simulink model "InverterModel"  (R2016a)
settings: Solver=FixedStepDiscrete  StartTime=0.0  StopTime=0.55e-6  FixedStep=SampleTime  RelTol=1e-3
values from neighbouring files (symbols this model uses):
  DelayTop = 0    [InverterMFile.m]
  Dtop = 48    [InverterMFile.m]
  fsw = 2000e3    (= 2000000)    [InverterMFile.m]
  Rd = 0.0024 + 1e-4    (= 0.0025)    [InverterMFile.m]
  Rg = 1.5    [InverterMFile.m]
  Rload = 20    [InverterMFile.m]    (also in TwoLevelSPWM-Hakan.m = Zload*Load_Power_Factor)
  Roff = 2    [InverterMFile.m]
  Ron = 15    [InverterMFile.m]
  Rs = 0.0433 + 1e-4    (= 0.0434)    [InverterMFile.m]
  Rss = 1e-3    (= 0.001)    [InverterMFile.m]
  VpulseMax = 6    [InverterMFile.m]
  VpulseMin = -3    [InverterMFile.m]
libraries: elec_lib x129, nesl_utility x91, fl_lib x80, simulink x6
(part 3 of 5)

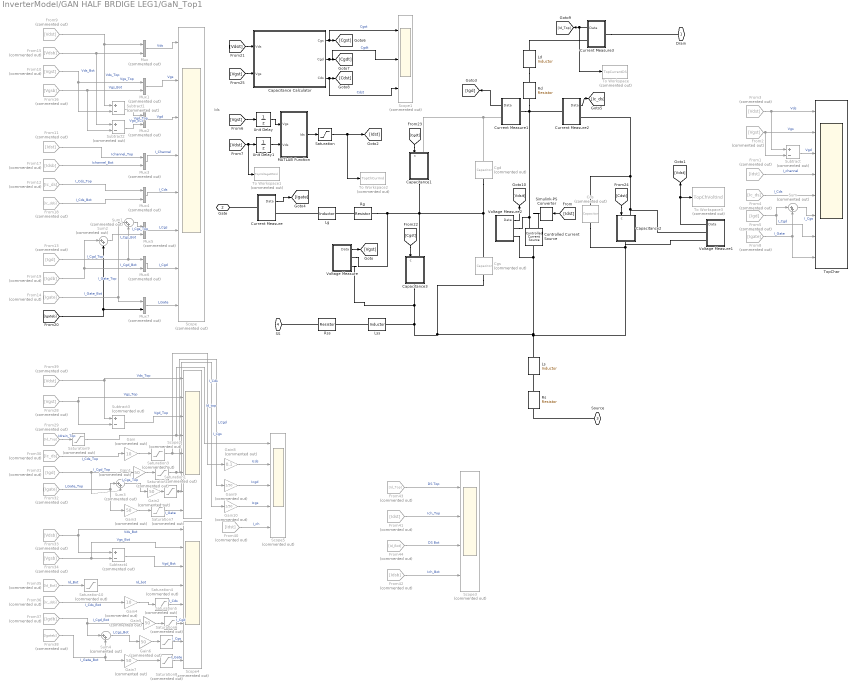
== system InverterModel/GAN HALF BRDIGE LEG1/GaN_Top1 ==
  note: Ids
  Capacitance Calculator : Subsystem
  Capacitance1 : Subsystem
  Capacitance2 : Subsystem
  Capacitance3 : Subsystem
  Cds : elec_lib/Passive Devices/Capacitor  Commented=on  enable_table=0  c=Cds F  Cvec=[ 1e-5 1e-6 ] F  Vvec=[ 0 10 ] V  CV_table_symmetry=1  C_tol=5  enable_C_tol=0  tol_distribution=1  nSigma=4  r=1e-6 Ohm  g=0 1/Ohm  initV=Vdc V  enable_operating_limits=0  operating_limit_action=2  max_working_voltage_range=[ -25 25 ] V  power_rating=1 W  enable_faults=0  fault_action=1  Cscale_faulted=100  R_faulted=0.001 Ohm  G_faulted=0 1/Ohm  tau_fault=0.001 s  enable_temporal_fault=0  t_fault=1 s  enable_behavioral_fault=0  max_permissible_voltage_range=[ -100 100 ] V  t_fail_on_voltage=1 s
  Cgd : elec_lib/Passive Devices/Capacitor  Commented=on  enable_table=0  c=Cgd F  Cvec=[ 1e-5 1e-6 ] F  Vvec=[ 0 10 ] V  CV_table_symmetry=1  C_tol=5  enable_C_tol=0  tol_distribution=1  nSigma=4  r=1e-6 Ohm  g=0 1/Ohm  initV=-VpulseMax V  enable_operating_limits=0  operating_limit_action=2  max_working_voltage_range=[ -25 25 ] V  power_rating=1 W  enable_faults=0  fault_action=1  Cscale_faulted=100  R_faulted=0.001 Ohm  G_faulted=0 1/Ohm  tau_fault=0.001 s  enable_temporal_fault=0  t_fault=1 s  enable_behavioral_fault=0  max_permissible_voltage_range=[ -100 100 ] V  t_fail_on_voltage=1 s
  Cgs : elec_lib/Passive Devices/Capacitor  Commented=on  enable_table=0  c=Cgs F  Cvec=[ 1e-5 1e-6 ] F  Vvec=[ 0 10 ] V  CV_table_symmetry=1  C_tol=5  enable_C_tol=0  tol_distribution=1  nSigma=4  r=1e-6 Ohm  g=0 1/Ohm  initV=VpulseMin V  enable_operating_limits=0  operating_limit_action=2  max_working_voltage_range=[ -25 25 ] V  power_rating=1 W  enable_faults=0  fault_action=1  Cscale_faulted=100  R_faulted=0.001 Ohm  G_faulted=0 1/Ohm  tau_fault=0.001 s  enable_temporal_fault=0  t_fault=1 s  enable_behavioral_fault=0  max_permissible_voltage_range=[ -100 100 ] V  t_fail_on_voltage=1 s
  Controlled Current Source : fl_lib/Electrical/Electrical Sources/Controlled Current Source
  Current Measure : Subsystem
  Current Measure1 : Subsystem
  Current Measure2 : Subsystem
  Current Measure3 : Subsystem
  From{1,11,40..41} (4 alike) : From  Commented=on  GotoTag=Idst  TagVisibility=global
  From10 : From  Commented=on  GotoTag=Vgst  TagVisibility=global
  From12 : From  Commented=on  GotoTag=Ic_ds
  From13 : From  Commented=on  GotoTag=Igd
  From14 : From  Commented=on  GotoTag=Igate
  From15 : From  Commented=on  GotoTag=Vdsb  TagVisibility=global
  From16 : From  Commented=on  GotoTag=Vgsb  TagVisibility=global
  From17 : From  Commented=on  GotoTag=Idsb  TagVisibility=global
  From18 : From  Commented=on  GotoTag=Ic_dsb  TagVisibility=global
  From19 : From  Commented=on  GotoTag=Igdb  TagVisibility=global
  From2 : From  Commented=on  GotoTag=Vgst  TagVisibility=global
  From28 : From  Commented=on  GotoTag=Vgst  TagVisibility=global
  From29 : From  Commented=on  GotoTag=Id_Top
  From3 : From  Commented=on  GotoTag=Vdst  TagVisibility=global
  From30 : From  Commented=on  GotoTag=Ic_ds
  From31 : From  Commented=on  GotoTag=Igd
  From32 : From  Commented=on  GotoTag=Igate
  From33 : From  Commented=on  GotoTag=Vdsb  TagVisibility=global
  From34 : From  Commented=on  GotoTag=Vgsb  TagVisibility=global
  From35 : From  Commented=on  GotoTag=Id_Bot  TagVisibility=global
  From36 : From  Commented=on  GotoTag=Ic_dsb  TagVisibility=global
  From37 : From  Commented=on  GotoTag=Igdb  TagVisibility=global
  From38 : From  Commented=on  GotoTag=Igateb  TagVisibility=global
  From39 : From  Commented=on  GotoTag=Vdst  TagVisibility=global
  From4 : From  Commented=on  GotoTag=Ic_ds
  From42 : From  Commented=on  GotoTag=Idsb  TagVisibility=global
  From43 : From  Commented=on  GotoTag=Id_Top
  From44 : From  Commented=on  GotoTag=Id_Bot  TagVisibility=global
  From5 : From  Commented=on  GotoTag=Igd
  From8 : From  Commented=on  GotoTag=Igate
  From9 : From  Commented=on  GotoTag=Vdst  TagVisibility=global
  Gain : Gain  Commented=on  Gain=10
  Gain{1..3,5..7} (6 alike) : Gain  Commented=on  Gain=50
  Gain10 : Gain  Commented=on  Gain=1/50
  Gain4 : Gain  Commented=on  Gain=10
  Gain8 : Gain  Commented=on  Gain=0.1
  Gain9 : Gain  Commented=on  Gain=1/50
  Ld : elec_lib/Passive Devices/Inductor  l=Ld H  L_tol=20  enable_L_tol=0  tol_distribution=1  nSigma=4  r=0 Ohm  g=1e-9 1/Ohm  initI=CurrBT A  enable_operating_limits=0  operating_limit_action=2  max_working_current=1 A  power_rating=1 W  enable_faults=0  fault_action=1  lambdaPercent=50  k_faulted=0.9999 Ohm  turnsShort=0  openCct=0  groundShort=0  groundShortG=0 1/Ohm  tau_fault=0.001 s  enable_temporal_fault=0  t_fault=1 s  enable_behavioral_fault=0  max_permissible_voltage=100 V  n_fail_on_voltage=1  max_permissible_current=1 A  t_fail_on_current=1 s
  Lg : elec_lib/Passive Devices/Inductor  l=Lg H  L_tol=20  enable_L_tol=0  tol_distribution=1  nSigma=4  r=0 Ohm  g=1e-9 1/Ohm  initI=0 A  enable_operating_limits=0  operating_limit_action=1  max_working_current=1 A  power_rating=1 W  enable_faults=0  fault_action=1  lambdaPercent=50  k_faulted=0.9999 Ohm  turnsShort=0  openCct=0  groundShort=0  groundShortG=0 1/Ohm  tau_fault=0.001 s  enable_temporal_fault=0  t_fault=1 s  enable_behavioral_fault=0  max_permissible_voltage=100 V  n_fail_on_voltage=1  max_permissible_current=1 A  t_fail_on_current=1 s
  Ls : elec_lib/Passive Devices/Inductor  l=Ls H  L_tol=20  enable_L_tol=0  tol_distribution=1  nSigma=4  r=0 Ohm  g=1e-9 1/Ohm  initI=CurrBT A  enable_operating_limits=0  operating_limit_action=2  max_working_current=1 A  power_rating=1 W  enable_faults=0  fault_action=1  lambdaPercent=50  k_faulted=0.9999 Ohm  turnsShort=0  openCct=0  groundShort=0  groundShortG=0 1/Ohm  tau_fault=0.001 s  enable_temporal_fault=0  t_fault=1 s  enable_behavioral_fault=0  max_permissible_voltage=100 V  n_fail_on_voltage=1  max_permissible_current=1 A  t_fail_on_current=1 s
  Lss : elec_lib/Passive Devices/Inductor  l=Lss H  L_tol=20  enable_L_tol=0  tol_distribution=1  nSigma=4  r=0 Ohm  g=1e-9 1/Ohm  initI=0 A  enable_operating_limits=0  operating_limit_action=2  max_working_current=1 A  power_rating=1 W  enable_faults=0  fault_action=1  lambdaPercent=50  k_faulted=0.9999 Ohm  turnsShort=0  openCct=0  groundShort=0  groundShortG=0 1/Ohm  tau_fault=0.001 s  enable_temporal_fault=0  t_fault=1 s  enable_behavioral_fault=0  max_permissible_voltage=100 V  n_fail_on_voltage=1  max_permissible_current=1 A  t_fail_on_current=1 s
  MATLAB Function : MATLAB Function  TreatAsAtomicUnit=on
  Mux{,1..7} (8 alike) : Mux  Commented=on  Inputs=2
  Rd : elec_lib/Passive Devices/Resistor  R=Rd Ohm  R_tol=5  enable_R_tol=0  tol_distribution=1  nSigma=4  enable_operating_limits=0  operating_limit_action=2  max_working_voltage=100 V  power_rating=1 W  enable_faults=0  fault_action=1  R_faulted=Inf Ohm  enable_temporal_fault=0  t_fault=1 s  enable_behavioral_fault=0  max_permissible_current=1 A  t_fail_on_current=1 s  noise_mode=0  sample_time=0.001 s  repeatability=1  auto_seed=2139298691  user_seed=0  Tdevice=25 degC  alpha=0.00393 1/K  Tmeas=25 degC  thermal_mass=100 J/K  initial_temperature=25 degC  power_derating_T1=70 degC  power_derating_T2=155 degC  operating_temperature_range_vec=[ -50 150 ] degC
  Rg : elec_lib/Passive Devices/Resistor  R=Rg Ohm  R_tol=5  enable_R_tol=0  tol_distribution=1  nSigma=4  enable_operating_limits=0  operating_limit_action=2  max_working_voltage=100 V  power_rating=1 W  enable_faults=0  fault_action=1  R_faulted=Inf Ohm  enable_temporal_fault=0  t_fault=1 s  enable_behavioral_fault=0  max_permissible_current=1 A  t_fail_on_current=1 s  noise_mode=0  sample_time=0.001 s  repeatability=1  auto_seed=3869131976  user_seed=0  Tdevice=25 degC  alpha=0.00393 1/K  Tmeas=25 degC  thermal_mass=100 J/K  initial_temperature=25 degC  power_derating_T1=70 degC  power_derating_T2=155 degC  operating_temperature_range_vec=[ -50 150 ] degC
  Rs : elec_lib/Passive Devices/Resistor  R=Rs Ohm  R_tol=5  enable_R_tol=0  tol_distribution=1  nSigma=4  enable_operating_limits=0  operating_limit_action=2  max_working_voltage=100 V  power_rating=1 W  enable_faults=0  fault_action=1  R_faulted=Inf Ohm  enable_temporal_fault=0  t_fault=1 s  enable_behavioral_fault=0  max_permissible_current=1 A  t_fail_on_current=1 s  noise_mode=0  sample_time=0.001 s  repeatability=1  auto_seed=2468151142  user_seed=0  Tdevice=25 degC  alpha=0.00393 1/K  Tmeas=25 degC  thermal_mass=100 J/K  initial_temperature=25 degC  power_derating_T1=70 degC  power_derating_T2=155 degC  operating_temperature_range_vec=[ -50 150 ] degC
  Rss : elec_lib/Passive Devices/Resistor  R=Rss Ohm  R_tol=5  enable_R_tol=0  tol_distribution=1  nSigma=4  enable_operating_limits=0  operating_limit_action=2  max_working_voltage=100 V  power_rating=1 W  enable_faults=0  fault_action=1  R_faulted=Inf Ohm  enable_temporal_fault=0  t_fault=1 s  enable_behavioral_fault=0  max_permissible_current=1 A  t_fail_on_current=1 s  noise_mode=0  sample_time=0.001 s  repeatability=1  auto_seed=3630012664  user_seed=0  Tdevice=25 degC  alpha=0.00393 1/K  Tmeas=25 degC  thermal_mass=100 J/K  initial_temperature=25 degC  power_derating_T1=70 degC  power_derating_T2=155 degC  operating_temperature_range_vec=[ -50 150 ] degC
  Saturation : Saturate  UpperLimit=200  LowerLimit=-200
  Saturation{1..2,5..10} (8 alike) : Saturate  Commented=on  UpperLimit=100  LowerLimit=-100
  Saturation3 : Saturate  Commented=on  UpperLimit=250  LowerLimit=-100
  Saturation4 : Saturate  Commented=on  UpperLimit=250  LowerLimit=-100
  Scope : Scope  Commented=on  NumInputPorts=8
  Scope1 : Scope  Commented=on  NumInputPorts=3
  Scope2 : Scope  Commented=on  NumInputPorts=8
  Scope3 : Scope  Commented=on  NumInputPorts=4
  Scope4 : Scope  Commented=on  NumInputPorts=8
  Scope5 : Scope  Commented=on  NumInputPorts=5
  Simulink-PS Converter : nesl_utility/Simulink-PS Converter  PhysicalDomain=network_engine_domain  SubClassName=ps_input  LeftPortType=input  RightPortType=output  PseudoPeriodic=off  Frequencies=[]  NoiseDistribution=none  NoiseParameters=[]  Unit=1  AffineConversion=off  InputFiltering=off  SimscapeFilterOrder=1  InputFilterTimeConstant=0.001  UdotUserProvided=1
  Subtract{,1..4} (5 alike) : Sum  Commented=on  Inputs=+-
  Sum{,1..4} (5 alike) : Sum  Commented=on  Inputs=|++
  To Workspace : ToWorkspace  Commented=on  VariableName=TopCurrentDS  SampleTime=-1
      settings: Save2DSignal=2-D array (concatenate along first dimension)
  To Workspace1 : ToWorkspace  Commented=on  VariableName=TopVoltageDSInd  SampleTime=-1
      settings: Save2DSignal=2-D array (concatenate along first dimension)
  To Workspace2 : ToWorkspace  Commented=on  VariableName=TopChCurrInd  SampleTime=-1
      settings: Save2DSignal=2-D array (concatenate along first dimension)
  To Workspace3 : ToWorkspace  Commented=on  VariableName=TopChVoltInd  SampleTime=-1
      settings: Save2DSignal=2-D array (concatenate along first dimension)
  TopChar : Scope  NumInputPorts=8
  Unit Delay : UnitDelay  SampleTime=-1
  Unit Delay1 : UnitDelay  SampleTime=-1
  Voltage Measure : Subsystem
  Voltage Measure1 : Subsystem
  Voltage Measure2 : Subsystem
  Drain : PMIOPort  Port=1  Side=Right
  Gate : PMIOPort  Port=2  Side=Left
  Source : PMIOPort  Port=3  Side=Right
  SS : PMIOPort  Port=4  Side=Left
  wires:
  [Vgst] -> Capacitance Calculator/2(Vgs)
  From44/1 -> Scope3/3  "DS Bot"
  From43/1 -> Scope3/1  "DS Top"
  Voltage Measure1/1(Data) -> [Vdst], To Workspace3/1
  Saturation/1 -> To Workspace2/1, [Idst]
  Voltage Measure2/1(Data) -> [Vdsit]
  Unit Delay1/1 -> MATLAB Function/2(Vds)
  [Vdst] -> To Workspace1/1, Unit Delay1/1
  From42/1 -> Scope3/4  "Ich_Bot"
  From41/1 -> Scope3/2  "Ich_Top"
  From40/1 -> Scope5/5  "I_ch"
  Gain10/1 -> Scope5/4  "Icgs"
  Gain9/1 -> Scope5/3  "Icgd"
  Gain8/1 -> Scope5/2  "Icds"
  Saturation10/1 -> Scope4/4  "Id_bot"
  Saturation9/1 -> Scope2/4, Scope5/1  "Id_top"
  Current Measure3/1(Data) -> [Id_Top], To Workspace/1
  Saturation8/1 -> Scope4/8  "I_Gate"
  Saturation7/1 -> Scope2/8  "I_Gate"
  Saturation6/1 -> Scope4/7  "I_Cgs"
  Gain5/1 -> Saturation5/1
  Saturation5/1 -> Scope4/6  "I_Cgd"
  Saturation4/1 -> Scope4/5  "I_Cds"
  Saturation3/1 -> Scope2/5, Gain8/1  "I_Cds"
  Saturation2/1 -> Scope2/6, Gain9/1  "I_Cgd"
  Saturation1/1 -> Scope2/7, Gain10/1  "I_Cgs"
  Gain2/1 -> Saturation1/1
  Gain7/1 -> Saturation8/1
  Gain6/1 -> Saturation6/1
  Gain4/1 -> Saturation4/1
  Gain3/1 -> Saturation7/1
  Sum3/1 -> Gain2/1  "I_Cgs_Top"
  Gain1/1 -> Saturation2/1
  Gain/1 -> Saturation3/1
  Sum4/1 -> Gain6/1  "I_Cgs_Bot"
  From35/1 -> Saturation10/1  "Id_Bot"
  From29/1 -> Saturation9/1  "Idrain_Top"
  Subtract4/1 -> Scope4/3  "Vgd_Bot"
  Subtract3/1 -> Scope2/3  "Vgd_Top"
  From38/1 -> Sum4/2, Gain7/1  "I_Gate_Bot"
  From37/1 -> Gain5/1, Sum4/1  "I_Cgd_Bot"
  From36/1 -> Gain4/1  "I_Cds_Bot"
  From34/1 -> Subtract4/2, Scope4/2  "Vgs_Bot"
  From33/1 -> Subtract4/1, Scope4/1  "Vds_Bot"
  From32/1 -> Sum3/1, Gain3/1  "I_Gate_Top"
  From31/1 -> Gain1/1, Sum3/2  "I_Cgd_Top"
  From30/1 -> Gain/1  "I_Cds_Top"
  From28/1 -> Subtract3/2, Scope2/2  "Vgs_Top"
  From39/1 -> Subtract3/1, Scope2/1  "Vds_Top"
  [Cdst] -> Capacitance2/1(c)
  [Cgdt] -> Capacitance1/1(c)
  [Cgst] -> Capacitance3/1(c)
  Capacitance Calculator/3(Cds) -> [Cdst], Scope1/3  "Cdst"
  Capacitance Calculator/2(Cgd) -> [Cgdt], Scope1/2  "Cgdt"
  Capacitance Calculator/1(Cgs) -> [Cgst], Scope1/1  "Cgst"
  [Vdsit] -> Capacitance Calculator/1(Vds)
  Mux/1 -> Scope/1  "Vds"
  Mux1/1 -> Scope/2  "Vgs"
  Mux2/1 -> Scope/3  "Vgd"
  Mux3/1 -> Scope/4  "I_Channel"
  Mux4/1 -> Scope/5  "I_Cds"
  Mux5/1 -> Scope/6  "I_Cgs"
  Mux6/1 -> Scope/7  "I_Cgd"
  Mux7/1 -> Scope/8  "I_Gate"
  From17/1 -> Mux3/2  "Ichannel_Bot"
  From11/1 -> Mux3/1  "Ichannel_Top"
  Subtract2/1 -> Mux2/2  "Vgd_Bot"
  Subtract1/1 -> Mux2/1  "Vgd_Top"
  Sum2/1 -> Mux5/2  "I_Cgs_Bot"
  [Igateb] -> Sum2/2, Mux7/2  "I_Gate_Bot"
  From19/1 -> Sum2/1, Mux6/2  "I_Cgd_Bot"
  From18/1 -> Mux4/2  "I_Cds_Bot"
  From16/1 -> Subtract2/2, Mux1/2  "Vgs_Bot"
  From15/1 -> Mux/2, Subtract2/1  "Vds_Bot"
  Sum1/1 -> Mux5/1  "I_Cgs_Top"
  From14/1 -> Sum1/1, Mux7/1  "I_Gate_Top"
  From13/1 -> Sum1/2, Mux6/1  "I_Cgd_Top"
  From12/1 -> Mux4/1  "I_Cds_Top"
  From10/1 -> Subtract1/2, Mux1/1  "Vgs_Top"
  From9/1 -> Subtract1/1, Mux/1  "Vds_Top"
  Voltage Measure/1(Data) -> [Vgst]
  Current Measure/1(Data) -> [Igate]
  Sum/1 -> TopChar/6  "I_Cgs"
  From4/1 -> TopChar/5  "I_Cds"
  From8/1 -> Sum/2, TopChar/8  "I_Gate"
  From5/1 -> Sum/1, TopChar/7  "I_Cgd"
  Current Measure2/1(Data) -> [Ic_ds]
  Current Measure1/1(Data) -> [Igd]
  Subtract/1 -> TopChar/3  "Vgd"
  From1/1 -> TopChar/4  "I_channel"
  From3/1 -> TopChar/1, Subtract/1  "Vds"
  From2/1 -> TopChar/2, Subtract/2  "Vgs"
  [Idst] -> Simulink-PS Converter/1
  Unit Delay/1 -> MATLAB Function/1(Vgs)
  MATLAB Function/1(Ids) -> Saturation/1
  [Vgst] -> Unit Delay/1
  connections:
  Rg/RConn1 -- Lg/RConn1
  Current Measure3/RConn1 -- Ld/LConn1
  Rs/LConn1 -- Ls/RConn1
  Lss/LConn1 -- Rss/RConn1
  Ld/RConn1 -- Rd/LConn1
  Source/RConn1 -- Rs/RConn1
  Voltage Measure/RConn2 -- Capacitance3/RConn1 -- Cgs/RConn1 -- Voltage Measure2/RConn2 -- Controlled Current Source/LConn1 -- Capacitance2/RConn1 -- Voltage Measure1/RConn2 -- Cds/RConn1 -- Ls/LConn1 -- Lss/RConn1
  Rss/LConn1 -- SS/RConn1
  Lg/LConn1 -- Current Measure/RConn1
  Current Measure1/LConn1 -- Rd/RConn1 -- Controlled Current Source/RConn2 -- Voltage Measure2/RConn1 -- Current Measure2/LConn1
  Current Measure3/LConn1 -- Drain/RConn1
  Current Measure2/RConn1 -- Cds/LConn1 -- Voltage Measure1/RConn1 -- Capacitance2/LConn1
  Cgd/LConn1 -- Current Measure1/RConn1 -- Capacitance1/LConn1
  Current Measure/LConn1 -- Gate/RConn1
  Simulink-PS Converter/RConn1 -- Controlled Current Source/RConn1
  Voltage Measure/RConn1 -- Rg/LConn1 -- Capacitance3/LConn1 -- Cgd/RConn1 -- Cgs/LConn1 -- Capacitance1/RConn1

== system InverterModel/GAN HALF BRDIGE LEG1/Voltage Measure3 ==
  PS-Simulink Converter2 : nesl_utility/PS-Simulink Converter  PhysicalDomain=network_engine_domain  SubClassName=ps_output  LeftPortType=input  RightPortType=output  PseudoPeriodic=off  Frequencies=[]  Unit=1  AffineConversion=off
  Voltage Sensor3 : fl_lib/Electrical/Electrical Sensors/Voltage Sensor
  V+ : PMIOPort  Port=1  Side=Right
  V- : PMIOPort  Port=2  Side=Right
  Data : Outport
  wires:
  PS-Simulink Converter2/1 -> Data/1
  connections:
  PS-Simulink Converter2/LConn1 -- Voltage Sensor3/RConn1
  Voltage Sensor3/RConn2 -- V-/RConn1
  Voltage Sensor3/LConn1 -- V+/RConn1

== system InverterModel/GAN HALF BRDIGE LEG1/Voltage Measure6 ==
  PS-Simulink Converter2 : nesl_utility/PS-Simulink Converter  PhysicalDomain=network_engine_domain  SubClassName=ps_output  LeftPortType=input  RightPortType=output  PseudoPeriodic=off  Frequencies=[]  Unit=1  AffineConversion=off
  Voltage Sensor3 : fl_lib/Electrical/Electrical Sensors/Voltage Sensor
  V+ : PMIOPort  Port=1  Side=Right
  V- : PMIOPort  Port=2  Side=Right
  Data : Outport
  wires:
  PS-Simulink Converter2/1 -> Data/1
  connections:
  Voltage Sensor3/LConn1 -- V+/RConn1
  Voltage Sensor3/RConn2 -- V-/RConn1
  PS-Simulink Converter2/LConn1 -- Voltage Sensor3/RConn1

== system InverterModel/GAN HALF BRDIGE LEG2/Current Measure4 ==
  Current Sensor1 : fl_lib/Electrical/Electrical Sensors/Current Sensor
  PS-Simulink Converter4 : nesl_utility/PS-Simulink Converter  PhysicalDomain=network_engine_domain  SubClassName=ps_output  LeftPortType=input  RightPortType=output  PseudoPeriodic=off  Frequencies=[]  Unit=1  AffineConversion=off
  I+ : PMIOPort  Port=1  Side=Left
  I- : PMIOPort  Port=2  Side=Right
  Data : Outport
  wires:
  PS-Simulink Converter4/1 -> Data/1
  connections:
  Current Sensor1/LConn1 -- I+/RConn1
  PS-Simulink Converter4/LConn1 -- Current Sensor1/RConn1
  Current Sensor1/RConn2 -- I-/RConn1

== system InverterModel/GAN HALF BRDIGE LEG2/Current Measure5 ==
  Current Sensor1 : fl_lib/Electrical/Electrical Sensors/Current Sensor
  PS-Simulink Converter4 : nesl_utility/PS-Simulink Converter  PhysicalDomain=network_engine_domain  SubClassName=ps_output  LeftPortType=input  RightPortType=output  PseudoPeriodic=off  Frequencies=[]  Unit=1  AffineConversion=off
  I+ : PMIOPort  Port=1  Side=Left
  I- : PMIOPort  Port=2  Side=Right
  Data : Outport
  wires:
  PS-Simulink Converter4/1 -> Data/1
  connections:
  Current Sensor1/RConn2 -- I-/RConn1
  PS-Simulink Converter4/LConn1 -- Current Sensor1/RConn1
  Current Sensor1/LConn1 -- I+/RConn1

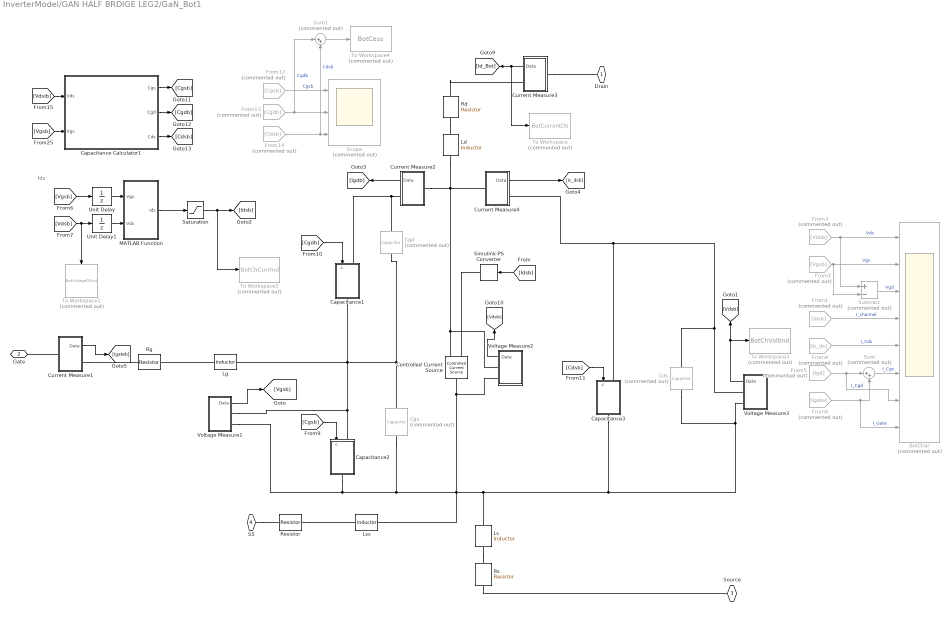
== system InverterModel/GAN HALF BRDIGE LEG2/GaN_Bot1 ==
  note: Ids
  BotChar : Scope  Commented=on  NumInputPorts=8
  Capacitance Calculator1 : Subsystem
  Capacitance1 : Subsystem
  Capacitance2 : Subsystem
  Capacitance3 : Subsystem
  Cds : elec_lib/Passive Devices/Capacitor  Commented=on  enable_table=0  c=Cds F  Cvec=[ 1e-5 1e-6 ] F  Vvec=[ 0 10 ] V  CV_table_symmetry=1  C_tol=5  enable_C_tol=0  tol_distribution=1  nSigma=4  r=1e-6 Ohm  g=0 1/Ohm  initV=0 V  enable_operating_limits=0  operating_limit_action=2  max_working_voltage_range=[ -25 25 ] V  power_rating=1 W  enable_faults=0  fault_action=1  Cscale_faulted=100  R_faulted=0.001 Ohm  G_faulted=0 1/Ohm  tau_fault=0.001 s  enable_temporal_fault=0  t_fault=1 s  enable_behavioral_fault=0  max_permissible_voltage_range=[ -100 100 ] V  t_fail_on_voltage=1 s
  Cgd : elec_lib/Passive Devices/Capacitor  Commented=on  enable_table=0  c=Cgd F  Cvec=[ 1e-5 1e-6 ] F  Vvec=[ 0 10 ] V  CV_table_symmetry=1  C_tol=5  enable_C_tol=0  tol_distribution=1  nSigma=4  r=1e-6 Ohm  g=0 1/Ohm  initV=Vdc - VpulseMin V  enable_operating_limits=0  operating_limit_action=2  max_working_voltage_range=[ -25 25 ] V  power_rating=1 W  enable_faults=0  fault_action=1  Cscale_faulted=100  R_faulted=0.001 Ohm  G_faulted=0 1/Ohm  tau_fault=0.001 s  enable_temporal_fault=0  t_fault=1 s  enable_behavioral_fault=0  max_permissible_voltage_range=[ -100 100 ] V  t_fail_on_voltage=1 s
  Cgs : elec_lib/Passive Devices/Capacitor  Commented=on  enable_table=0  c=Cgs F  Cvec=[ 1e-5 1e-6 ] F  Vvec=[ 0 10 ] V  CV_table_symmetry=1  C_tol=5  enable_C_tol=0  tol_distribution=1  nSigma=4  r=1e-6 Ohm  g=0 1/Ohm  initV=VpulseMax V  enable_operating_limits=0  operating_limit_action=2  max_working_voltage_range=[ -25 25 ] V  power_rating=1 W  enable_faults=0  fault_action=1  Cscale_faulted=100  R_faulted=0.001 Ohm  G_faulted=0 1/Ohm  tau_fault=0.001 s  enable_temporal_fault=0  t_fault=1 s  enable_behavioral_fault=0  max_permissible_voltage_range=[ -100 100 ] V  t_fail_on_voltage=1 s
  Controlled Current Source : fl_lib/Electrical/Electrical Sources/Controlled Current Source
  Current Measure1 : Subsystem
  Current Measure2 : Subsystem
  Current Measure3 : Subsystem
  Current Measure4 : Subsystem
  From1 : From  Commented=on  GotoTag=Idsb  TagVisibility=global
  From12 : From  Commented=on  GotoTag=Cgsb
  From13 : From  Commented=on  GotoTag=Cgdb
  From14 : From  Commented=on  GotoTag=Cdsb
  From2 : From  Commented=on  GotoTag=Vgsb  TagVisibility=global
  From3 : From  Commented=on  GotoTag=Vdsb  TagVisibility=global
  From4 : From  Commented=on  GotoTag=Ic_ds
  From5 : From  Commented=on  GotoTag=Igd
  From8 : From  Commented=on  GotoTag=Igate
  Ld : elec_lib/Passive Devices/Inductor  l=Ld H  L_tol=20  enable_L_tol=0  tol_distribution=1  nSigma=4  r=0 Ohm  g=1e-9 1/Ohm  initI=CurrCB A  enable_operating_limits=0  operating_limit_action=2  max_working_current=1 A  power_rating=1 W  enable_faults=0  fault_action=1  lambdaPercent=50  k_faulted=0.9999 Ohm  turnsShort=0  openCct=0  groundShort=0  groundShortG=0 1/Ohm  tau_fault=0.001 s  enable_temporal_fault=0  t_fault=1 s  enable_behavioral_fault=0  max_permissible_voltage=100 V  n_fail_on_voltage=1  max_permissible_current=1 A  t_fail_on_current=1 s
  "Lg " : elec_lib/Passive Devices/Inductor  l=Lg H  L_tol=20  enable_L_tol=0  tol_distribution=1  nSigma=4  r=0 Ohm  g=1e-9 1/Ohm  initI=0 A  enable_operating_limits=0  operating_limit_action=2  max_working_current=1 A  power_rating=1 W  enable_faults=0  fault_action=1  lambdaPercent=50  k_faulted=0.9999 Ohm  turnsShort=0  openCct=0  groundShort=0  groundShortG=0 1/Ohm  tau_fault=0.001 s  enable_temporal_fault=0  t_fault=1 s  enable_behavioral_fault=0  max_permissible_voltage=100 V  n_fail_on_voltage=1  max_permissible_current=1 A  t_fail_on_current=1 s
  Ls : elec_lib/Passive Devices/Inductor  l=Ls H  L_tol=20  enable_L_tol=0  tol_distribution=1  nSigma=4  r=0 Ohm  g=1e-9 1/Ohm  initI=CurrCB A  enable_operating_limits=0  operating_limit_action=2  max_working_current=1 A  power_rating=1 W  enable_faults=0  fault_action=1  lambdaPercent=50  k_faulted=0.9999 Ohm  turnsShort=0  openCct=0  groundShort=0  groundShortG=0 1/Ohm  tau_fault=0.001 s  enable_temporal_fault=0  t_fault=1 s  enable_behavioral_fault=0  max_permissible_voltage=100 V  n_fail_on_voltage=1  max_permissible_current=1 A  t_fail_on_current=1 s
  Lss : elec_lib/Passive Devices/Inductor  l=Lss H  L_tol=20  enable_L_tol=0  tol_distribution=1  nSigma=4  r=0 Ohm  g=1e-9 1/Ohm  initI=0 A  enable_operating_limits=0  operating_limit_action=1  max_working_current=1 A  power_rating=1 W  enable_faults=0  fault_action=1  lambdaPercent=50  k_faulted=0.9999 Ohm  turnsShort=0  openCct=0  groundShort=0  groundShortG=0 1/Ohm  tau_fault=0.001 s  enable_temporal_fault=0  t_fault=1 s  enable_behavioral_fault=0  max_permissible_voltage=100 V  n_fail_on_voltage=1  max_permissible_current=1 A  t_fail_on_current=1 s
  MATLAB Function : MATLAB Function  TreatAsAtomicUnit=on
  Rd : elec_lib/Passive Devices/Resistor  R=Rd Ohm  R_tol=5  enable_R_tol=0  tol_distribution=1  nSigma=4  enable_operating_limits=0  operating_limit_action=2  max_working_voltage=100 V  power_rating=1 W  enable_faults=0  fault_action=1  R_faulted=Inf Ohm  enable_temporal_fault=0  t_fault=1 s  enable_behavioral_fault=0  max_permissible_current=1 A  t_fail_on_current=1 s  noise_mode=0  sample_time=0.001 s  repeatability=1  auto_seed=3172435897  user_seed=0  Tdevice=25 degC  alpha=0.00393 1/K  Tmeas=25 degC  thermal_mass=100 J/K  initial_temperature=25 degC  power_derating_T1=70 degC  power_derating_T2=155 degC  operating_temperature_range_vec=[ -50 150 ] degC
  Resistor : elec_lib/Passive Devices/Resistor  R=Rss Ohm  R_tol=5  enable_R_tol=0  tol_distribution=1  nSigma=4  enable_operating_limits=0  operating_limit_action=2  max_working_voltage=100 V  power_rating=1 W  enable_faults=0  fault_action=1  R_faulted=Inf Ohm  enable_temporal_fault=0  t_fault=1 s  enable_behavioral_fault=0  max_permissible_current=1 A  t_fail_on_current=1 s  noise_mode=0  sample_time=0.001 s  repeatability=1  auto_seed=2516795155  user_seed=0  Tdevice=25 degC  alpha=0.00393 1/K  Tmeas=25 degC  thermal_mass=100 J/K  initial_temperature=25 degC  power_derating_T1=70 degC  power_derating_T2=155 degC  operating_temperature_range_vec=[ -50 150 ] degC
  Rg : elec_lib/Passive Devices/Resistor  R=Rg Ohm  R_tol=5  enable_R_tol=0  tol_distribution=1  nSigma=4  enable_operating_limits=0  operating_limit_action=2  max_working_voltage=100 V  power_rating=1 W  enable_faults=0  fault_action=1  R_faulted=Inf Ohm  enable_temporal_fault=0  t_fault=1 s  enable_behavioral_fault=0  max_permissible_current=1 A  t_fail_on_current=1 s  noise_mode=0  sample_time=0.001 s  repeatability=1  auto_seed=1059716720  user_seed=0  Tdevice=25 degC  alpha=0.00393 1/K  Tmeas=25 degC  thermal_mass=100 J/K  initial_temperature=25 degC  power_derating_T1=70 degC  power_derating_T2=155 degC  operating_temperature_range_vec=[ -50 150 ] degC
  Rs : elec_lib/Passive Devices/Resistor  R=Rs Ohm  R_tol=5  enable_R_tol=0  tol_distribution=1  nSigma=4  enable_operating_limits=0  operating_limit_action=2  max_working_voltage=100 V  power_rating=1 W  enable_faults=0  fault_action=1  R_faulted=Inf Ohm  enable_temporal_fault=0  t_fault=1 s  enable_behavioral_fault=0  max_permissible_current=1 A  t_fail_on_current=1 s  noise_mode=0  sample_time=0.001 s  repeatability=1  auto_seed=2862235859  user_seed=0  Tdevice=25 degC  alpha=0.00393 1/K  Tmeas=25 degC  thermal_mass=100 J/K  initial_temperature=25 degC  power_derating_T1=70 degC  power_derating_T2=155 degC  operating_temperature_range_vec=[ -50 150 ] degC
  Saturation : Saturate  UpperLimit=200  LowerLimit=-200
  Scope : Scope  Commented=on  NumInputPorts=3
  Simulink-PS Converter : nesl_utility/Simulink-PS Converter  PhysicalDomain=network_engine_domain  SubClassName=ps_input  LeftPortType=input  RightPortType=output  PseudoPeriodic=off  Frequencies=[]  NoiseDistribution=none  NoiseParameters=[]  Unit=1  AffineConversion=off  InputFiltering=off  SimscapeFilterOrder=1  InputFilterTimeConstant=0.001  UdotUserProvided=1
  Subtract : Sum  Commented=on  Inputs=+-
  Sum : Sum  Commented=on  Inputs=|++
  Sum1 : Sum  Commented=on  Inputs=|++
  To Workspace : ToWorkspace  Commented=on  VariableName=BotCurrentDS  SampleTime=-1
      settings: Save2DSignal=2-D array (concatenate along first dimension)
  To Workspace1 : ToWorkspace  Commented=on  VariableName=BotVoltageDSInd  SampleTime=-1
      settings: Save2DSignal=2-D array (concatenate along first dimension)
  To Workspace2 : ToWorkspace  Commented=on  VariableName=BotChCurrInd  SampleTime=-1
      settings: Save2DSignal=2-D array (concatenate along first dimension)
  To Workspace3 : ToWorkspace  Commented=on  VariableName=BotChVoltInd  SampleTime=-1
      settings: Save2DSignal=2-D array (concatenate along first dimension)
  To Workspace4 : ToWorkspace  Commented=on  VariableName=BotCoss  SampleTime=-1
      settings: Save2DSignal=2-D array (concatenate along first dimension)
  Unit Delay : UnitDelay  SampleTime=-1
  Unit Delay1 : UnitDelay  SampleTime=-1
  Voltage Measure1 : Subsystem
  Voltage Measure2 : Subsystem
  Voltage Measure3 : Subsystem
  Drain : PMIOPort  Port=1  Side=Right
  Gate : PMIOPort  Port=2  Side=Left
  Source : PMIOPort  Port=3  Side=Right
  SS : PMIOPort  Port=4  Side=Left
  wires:
  Sum1/1 -> To Workspace4/1
  [Vgsb] -> Capacitance Calculator1/2(Vgs)
  Capacitance Calculator1/3(Cds) -> [Cdsb]
  Capacitance Calculator1/2(Cgd) -> [Cgdb]
  Capacitance Calculator1/1(Cgs) -> [Cgsb]
  [Vdsib] -> Capacitance Calculator1/1(Vds)
  Saturation/1 -> To Workspace2/1, [Idsb]
  Voltage Measure2/1(Data) -> [Vdsib]
  Unit Delay1/1 -> MATLAB Function/2(Vds)
  Current Measure3/1(Data) -> [Id_Bot], To Workspace/1
  From14/1 -> Scope/3, Sum1/2  "Cdsb"
  From13/1 -> Scope/2, Sum1/1  "Cgdb"
  From12/1 -> Scope/1  "Cgsb"
  [Cdsb] -> Capacitance3/1(c)
  [Cgdb] -> Capacitance1/1(c)
  [Cgsb] -> Capacitance2/1(c)
  Voltage Measure3/1(Data) -> [Vdsb], To Workspace3/1
  Current Measure1/1(Data) -> [Igateb]
  Sum/1 -> BotChar/6  "I_Cgs"
  Current Measure4/1(Data) -> [Ic_dsb]
  Current Measure2/1(Data) -> [Igdb]
  From8/1 -> Sum/2, BotChar/8  "I_Gate"
  From5/1 -> Sum/1, BotChar/7  "I_Cgd"
  From4/1 -> BotChar/5  "I_Cds"
  Subtract/1 -> BotChar/3  "Vgd"
  From1/1 -> BotChar/4  "I_channel"
  From3/1 -> Subtract/1, BotChar/1  "Vds"
  From2/1 -> Subtract/2, BotChar/2  "Vgs"
  [Idsb] -> Simulink-PS Converter/1
  [Vgsb] -> Unit Delay/1
  MATLAB Function/1(Ids) -> Saturation/1
  Unit Delay/1 -> MATLAB Function/1(Vgs)
  [Vdsb] -> To Workspace1/1, Unit Delay1/1
  Voltage Measure1/1(Data) -> [Vgsb]
  connections:
  Ls/RConn1 -- Rs/LConn1
  "Lg "/LConn1 -- Rg/LConn1
  Rd/RConn1 -- Ld/LConn1
  Resistor/RConn1 -- Lss/LConn1
  Rd/LConn1 -- Current Measure3/RConn1
  Rs/RConn1 -- Source/RConn1
  Voltage Measure3/RConn2 -- Cgs/RConn1 -- Capacitance2/RConn1 -- Voltage Measure1/RConn2 -- Voltage Measure2/RConn2 -- Controlled Current Source/LConn1 -- Lss/RConn1 -- Ls/LConn1 -- Capacitance3/RConn1 -- Cds/RConn1
  SS/RConn1 -- Resistor/LConn1
  Current Measure4/LConn1 -- Current Measure2/LConn1 -- Ld/RConn1 -- Voltage Measure2/RConn1 -- Controlled Current Source/RConn2
  Capacitance1/RConn1 -- Cgs/LConn1 -- Cgd/RConn1 -- "Lg "/RConn1 -- Voltage Measure1/RConn1 -- Capacitance2/LConn1
  Current Measure3/LConn1 -- Drain/RConn1
  Current Measure2/RConn1 -- Cgd/LConn1 -- Capacitance1/LConn1
  Current Measure1/RConn1 -- Rg/RConn1
  Current Measure4/RConn1 -- Capacitance3/LConn1 -- Cds/LConn1 -- Voltage Measure3/RConn1
  Current Measure1/LConn1 -- Gate/RConn1
  Simulink-PS Converter/RConn1 -- Controlled Current Source/RConn1

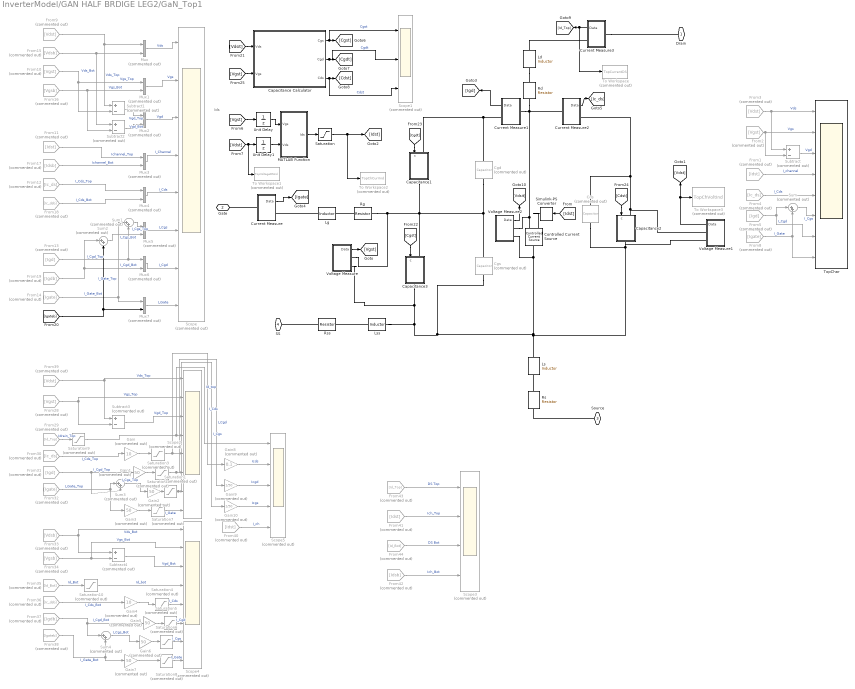
== system InverterModel/GAN HALF BRDIGE LEG2/GaN_Top1 ==
  note: Ids
  Capacitance Calculator : Subsystem
  Capacitance1 : Subsystem
  Capacitance2 : Subsystem
  Capacitance3 : Subsystem
  Cds : elec_lib/Passive Devices/Capacitor  Commented=on  enable_table=0  c=Cds F  Cvec=[ 1e-5 1e-6 ] F  Vvec=[ 0 10 ] V  CV_table_symmetry=1  C_tol=5  enable_C_tol=0  tol_distribution=1  nSigma=4  r=1e-6 Ohm  g=0 1/Ohm  initV=Vdc V  enable_operating_limits=0  operating_limit_action=2  max_working_voltage_range=[ -25 25 ] V  power_rating=1 W  enable_faults=0  fault_action=1  Cscale_faulted=100  R_faulted=0.001 Ohm  G_faulted=0 1/Ohm  tau_fault=0.001 s  enable_temporal_fault=0  t_fault=1 s  enable_behavioral_fault=0  max_permissible_voltage_range=[ -100 100 ] V  t_fail_on_voltage=1 s
  Cgd : elec_lib/Passive Devices/Capacitor  Commented=on  enable_table=0  c=Cgd F  Cvec=[ 1e-5 1e-6 ] F  Vvec=[ 0 10 ] V  CV_table_symmetry=1  C_tol=5  enable_C_tol=0  tol_distribution=1  nSigma=4  r=1e-6 Ohm  g=0 1/Ohm  initV=-VpulseMax V  enable_operating_limits=0  operating_limit_action=2  max_working_voltage_range=[ -25 25 ] V  power_rating=1 W  enable_faults=0  fault_action=1  Cscale_faulted=100  R_faulted=0.001 Ohm  G_faulted=0 1/Ohm  tau_fault=0.001 s  enable_temporal_fault=0  t_fault=1 s  enable_behavioral_fault=0  max_permissible_voltage_range=[ -100 100 ] V  t_fail_on_voltage=1 s
  Cgs : elec_lib/Passive Devices/Capacitor  Commented=on  enable_table=0  c=Cgs F  Cvec=[ 1e-5 1e-6 ] F  Vvec=[ 0 10 ] V  CV_table_symmetry=1  C_tol=5  enable_C_tol=0  tol_distribution=1  nSigma=4  r=1e-6 Ohm  g=0 1/Ohm  initV=VpulseMin V  enable_operating_limits=0  operating_limit_action=2  max_working_voltage_range=[ -25 25 ] V  power_rating=1 W  enable_faults=0  fault_action=1  Cscale_faulted=100  R_faulted=0.001 Ohm  G_faulted=0 1/Ohm  tau_fault=0.001 s  enable_temporal_fault=0  t_fault=1 s  enable_behavioral_fault=0  max_permissible_voltage_range=[ -100 100 ] V  t_fail_on_voltage=1 s
  Controlled Current Source : fl_lib/Electrical/Electrical Sources/Controlled Current Source
  Current Measure : Subsystem
  Current Measure1 : Subsystem
  Current Measure2 : Subsystem
  Current Measure3 : Subsystem
  From{1,11,40..41} (4 alike) : From  Commented=on  GotoTag=Idst  TagVisibility=global
  From10 : From  Commented=on  GotoTag=Vgst  TagVisibility=global
  From12 : From  Commented=on  GotoTag=Ic_ds
  From13 : From  Commented=on  GotoTag=Igd
  From14 : From  Commented=on  GotoTag=Igate
  From15 : From  Commented=on  GotoTag=Vdsb  TagVisibility=global
  From16 : From  Commented=on  GotoTag=Vgsb  TagVisibility=global
  From17 : From  Commented=on  GotoTag=Idsb  TagVisibility=global
  From18 : From  Commented=on  GotoTag=Ic_dsb  TagVisibility=global
  From19 : From  Commented=on  GotoTag=Igdb  TagVisibility=global
  From2 : From  Commented=on  GotoTag=Vgst  TagVisibility=global
  From28 : From  Commented=on  GotoTag=Vgst  TagVisibility=global
  From29 : From  Commented=on  GotoTag=Id_Top
  From3 : From  Commented=on  GotoTag=Vdst  TagVisibility=global
  From30 : From  Commented=on  GotoTag=Ic_ds
  From31 : From  Commented=on  GotoTag=Igd
  From32 : From  Commented=on  GotoTag=Igate
  From33 : From  Commented=on  GotoTag=Vdsb  TagVisibility=global
  From34 : From  Commented=on  GotoTag=Vgsb  TagVisibility=global
  From35 : From  Commented=on  GotoTag=Id_Bot  TagVisibility=global
  From36 : From  Commented=on  GotoTag=Ic_dsb  TagVisibility=global
  From37 : From  Commented=on  GotoTag=Igdb  TagVisibility=global
  From38 : From  Commented=on  GotoTag=Igateb  TagVisibility=global
  From39 : From  Commented=on  GotoTag=Vdst  TagVisibility=global
  From4 : From  Commented=on  GotoTag=Ic_ds
  From42 : From  Commented=on  GotoTag=Idsb  TagVisibility=global
  From43 : From  Commented=on  GotoTag=Id_Top
  From44 : From  Commented=on  GotoTag=Id_Bot  TagVisibility=global
  From5 : From  Commented=on  GotoTag=Igd
  From8 : From  Commented=on  GotoTag=Igate
  From9 : From  Commented=on  GotoTag=Vdst  TagVisibility=global
  Gain : Gain  Commented=on  Gain=10
  Gain{1..3,5..7} (6 alike) : Gain  Commented=on  Gain=50
  Gain10 : Gain  Commented=on  Gain=1/50
  Gain4 : Gain  Commented=on  Gain=10
  Gain8 : Gain  Commented=on  Gain=0.1
  Gain9 : Gain  Commented=on  Gain=1/50
  Ld : elec_lib/Passive Devices/Inductor  l=Ld H  L_tol=20  enable_L_tol=0  tol_distribution=1  nSigma=4  r=0 Ohm  g=1e-9 1/Ohm  initI=CurrCT A  enable_operating_limits=0  operating_limit_action=2  max_working_current=1 A  power_rating=1 W  enable_faults=0  fault_action=1  lambdaPercent=50  k_faulted=0.9999 Ohm  turnsShort=0  openCct=0  groundShort=0  groundShortG=0 1/Ohm  tau_fault=0.001 s  enable_temporal_fault=0  t_fault=1 s  enable_behavioral_fault=0  max_permissible_voltage=100 V  n_fail_on_voltage=1  max_permissible_current=1 A  t_fail_on_current=1 s
  Lg : elec_lib/Passive Devices/Inductor  l=Lg H  L_tol=20  enable_L_tol=0  tol_distribution=1  nSigma=4  r=0 Ohm  g=1e-9 1/Ohm  initI=0 A  enable_operating_limits=0  operating_limit_action=1  max_working_current=1 A  power_rating=1 W  enable_faults=0  fault_action=1  lambdaPercent=50  k_faulted=0.9999 Ohm  turnsShort=0  openCct=0  groundShort=0  groundShortG=0 1/Ohm  tau_fault=0.001 s  enable_temporal_fault=0  t_fault=1 s  enable_behavioral_fault=0  max_permissible_voltage=100 V  n_fail_on_voltage=1  max_permissible_current=1 A  t_fail_on_current=1 s
  Ls : elec_lib/Passive Devices/Inductor  l=Ls H  L_tol=20  enable_L_tol=0  tol_distribution=1  nSigma=4  r=0 Ohm  g=1e-9 1/Ohm  initI=CurrCT A  enable_operating_limits=0  operating_limit_action=2  max_working_current=1 A  power_rating=1 W  enable_faults=0  fault_action=1  lambdaPercent=50  k_faulted=0.9999 Ohm  turnsShort=0  openCct=0  groundShort=0  groundShortG=0 1/Ohm  tau_fault=0.001 s  enable_temporal_fault=0  t_fault=1 s  enable_behavioral_fault=0  max_permissible_voltage=100 V  n_fail_on_voltage=1  max_permissible_current=1 A  t_fail_on_current=1 s
  Lss : elec_lib/Passive Devices/Inductor  l=Lss H  L_tol=20  enable_L_tol=0  tol_distribution=1  nSigma=4  r=0 Ohm  g=1e-9 1/Ohm  initI=0 A  enable_operating_limits=0  operating_limit_action=2  max_working_current=1 A  power_rating=1 W  enable_faults=0  fault_action=1  lambdaPercent=50  k_faulted=0.9999 Ohm  turnsShort=0  openCct=0  groundShort=0  groundShortG=0 1/Ohm  tau_fault=0.001 s  enable_temporal_fault=0  t_fault=1 s  enable_behavioral_fault=0  max_permissible_voltage=100 V  n_fail_on_voltage=1  max_permissible_current=1 A  t_fail_on_current=1 s
  MATLAB Function : MATLAB Function  TreatAsAtomicUnit=on
  Mux{,1..7} (8 alike) : Mux  Commented=on  Inputs=2
  Rd : elec_lib/Passive Devices/Resistor  R=Rd Ohm  R_tol=5  enable_R_tol=0  tol_distribution=1  nSigma=4  enable_operating_limits=0  operating_limit_action=2  max_working_voltage=100 V  power_rating=1 W  enable_faults=0  fault_action=1  R_faulted=Inf Ohm  enable_temporal_fault=0  t_fault=1 s  enable_behavioral_fault=0  max_permissible_current=1 A  t_fail_on_current=1 s  noise_mode=0  sample_time=0.001 s  repeatability=1  auto_seed=358555955  user_seed=0  Tdevice=25 degC  alpha=0.00393 1/K  Tmeas=25 degC  thermal_mass=100 J/K  initial_temperature=25 degC  power_derating_T1=70 degC  power_derating_T2=155 degC  operating_temperature_range_vec=[ -50 150 ] degC
  Rg : elec_lib/Passive Devices/Resistor  R=Rg Ohm  R_tol=5  enable_R_tol=0  tol_distribution=1  nSigma=4  enable_operating_limits=0  operating_limit_action=2  max_working_voltage=100 V  power_rating=1 W  enable_faults=0  fault_action=1  R_faulted=Inf Ohm  enable_temporal_fault=0  t_fault=1 s  enable_behavioral_fault=0  max_permissible_current=1 A  t_fail_on_current=1 s  noise_mode=0  sample_time=0.001 s  repeatability=1  auto_seed=2688476806  user_seed=0  Tdevice=25 degC  alpha=0.00393 1/K  Tmeas=25 degC  thermal_mass=100 J/K  initial_temperature=25 degC  power_derating_T1=70 degC  power_derating_T2=155 degC  operating_temperature_range_vec=[ -50 150 ] degC
  Rs : elec_lib/Passive Devices/Resistor  R=Rs Ohm  R_tol=5  enable_R_tol=0  tol_distribution=1  nSigma=4  enable_operating_limits=0  operating_limit_action=2  max_working_voltage=100 V  power_rating=1 W  enable_faults=0  fault_action=1  R_faulted=Inf Ohm  enable_temporal_fault=0  t_fault=1 s  enable_behavioral_fault=0  max_permissible_current=1 A  t_fail_on_current=1 s  noise_mode=0  sample_time=0.001 s  repeatability=1  auto_seed=2838735261  user_seed=0  Tdevice=25 degC  alpha=0.00393 1/K  Tmeas=25 degC  thermal_mass=100 J/K  initial_temperature=25 degC  power_derating_T1=70 degC  power_derating_T2=155 degC  operating_temperature_range_vec=[ -50 150 ] degC
  Rss : elec_lib/Passive Devices/Resistor  R=Rss Ohm  R_tol=5  enable_R_tol=0  tol_distribution=1  nSigma=4  enable_operating_limits=0  operating_limit_action=2  max_working_voltage=100 V  power_rating=1 W  enable_faults=0  fault_action=1  R_faulted=Inf Ohm  enable_temporal_fault=0  t_fault=1 s  enable_behavioral_fault=0  max_permissible_current=1 A  t_fail_on_current=1 s  noise_mode=0  sample_time=0.001 s  repeatability=1  auto_seed=3134260353  user_seed=0  Tdevice=25 degC  alpha=0.00393 1/K  Tmeas=25 degC  thermal_mass=100 J/K  initial_temperature=25 degC  power_derating_T1=70 degC  power_derating_T2=155 degC  operating_temperature_range_vec=[ -50 150 ] degC
  Saturation : Saturate  UpperLimit=200  LowerLimit=-200
  Saturation{1..2,5..10} (8 alike) : Saturate  Commented=on  UpperLimit=100  LowerLimit=-100
  Saturation3 : Saturate  Commented=on  UpperLimit=250  LowerLimit=-100
  Saturation4 : Saturate  Commented=on  UpperLimit=250  LowerLimit=-100
  Scope : Scope  Commented=on  NumInputPorts=8
  Scope1 : Scope  Commented=on  NumInputPorts=3
  Scope2 : Scope  Commented=on  NumInputPorts=8
  Scope3 : Scope  Commented=on  NumInputPorts=4
  Scope4 : Scope  Commented=on  NumInputPorts=8
  Scope5 : Scope  Commented=on  NumInputPorts=5
  Simulink-PS Converter : nesl_utility/Simulink-PS Converter  PhysicalDomain=network_engine_domain  SubClassName=ps_input  LeftPortType=input  RightPortType=output  PseudoPeriodic=off  Frequencies=[]  NoiseDistribution=none  NoiseParameters=[]  Unit=1  AffineConversion=off  InputFiltering=off  SimscapeFilterOrder=1  InputFilterTimeConstant=0.001  UdotUserProvided=1
  Subtract{,1..4} (5 alike) : Sum  Commented=on  Inputs=+-
  Sum{,1..4} (5 alike) : Sum  Commented=on  Inputs=|++
  To Workspace : ToWorkspace  Commented=on  VariableName=TopCurrentDS  SampleTime=-1
      settings: Save2DSignal=2-D array (concatenate along first dimension)
  To Workspace1 : ToWorkspace  Commented=on  VariableName=TopVoltageDSInd  SampleTime=-1
      settings: Save2DSignal=2-D array (concatenate along first dimension)
  To Workspace2 : ToWorkspace  Commented=on  VariableName=TopChCurrInd  SampleTime=-1
      settings: Save2DSignal=2-D array (concatenate along first dimension)
  To Workspace3 : ToWorkspace  Commented=on  VariableName=TopChVoltInd  SampleTime=-1
      settings: Save2DSignal=2-D array (concatenate along first dimension)
  TopChar : Scope  NumInputPorts=8
  Unit Delay : UnitDelay  SampleTime=-1
  Unit Delay1 : UnitDelay  SampleTime=-1
  Voltage Measure : Subsystem
  Voltage Measure1 : Subsystem
  Voltage Measure2 : Subsystem
  Drain : PMIOPort  Port=1  Side=Right
  Gate : PMIOPort  Port=2  Side=Left
  Source : PMIOPort  Port=3  Side=Right
  SS : PMIOPort  Port=4  Side=Left
  wires:
  [Vgst] -> Unit Delay/1
  MATLAB Function/1(Ids) -> Saturation/1
  Unit Delay/1 -> MATLAB Function/1(Vgs)
  [Idst] -> Simulink-PS Converter/1
  From2/1 -> Subtract/2, TopChar/2  "Vgs"
  From3/1 -> Subtract/1, TopChar/1  "Vds"
  From1/1 -> TopChar/4  "I_channel"
  Subtract/1 -> TopChar/3  "Vgd"
  Current Measure1/1(Data) -> [Igd]
  Current Measure2/1(Data) -> [Ic_ds]
  From5/1 -> TopChar/7, Sum/1  "I_Cgd"
  From8/1 -> TopChar/8, Sum/2  "I_Gate"
  From4/1 -> TopChar/5  "I_Cds"
  Sum/1 -> TopChar/6  "I_Cgs"
  Current Measure/1(Data) -> [Igate]
  Voltage Measure/1(Data) -> [Vgst]
  From9/1 -> Mux/1, Subtract1/1  "Vds_Top"
  From10/1 -> Mux1/1, Subtract1/2  "Vgs_Top"
  From12/1 -> Mux4/1  "I_Cds_Top"
  From13/1 -> Mux6/1, Sum1/2  "I_Cgd_Top"
  From14/1 -> Mux7/1, Sum1/1  "I_Gate_Top"
  Sum1/1 -> Mux5/1  "I_Cgs_Top"
  From15/1 -> Subtract2/1, Mux/2  "Vds_Bot"
  From16/1 -> Mux1/2, Subtract2/2  "Vgs_Bot"
  From18/1 -> Mux4/2  "I_Cds_Bot"
  From19/1 -> Mux6/2, Sum2/1  "I_Cgd_Bot"
  [Igateb] -> Mux7/2, Sum2/2  "I_Gate_Bot"
  Sum2/1 -> Mux5/2  "I_Cgs_Bot"
  Subtract1/1 -> Mux2/1  "Vgd_Top"
  Subtract2/1 -> Mux2/2  "Vgd_Bot"
  From11/1 -> Mux3/1  "Ichannel_Top"
  From17/1 -> Mux3/2  "Ichannel_Bot"
  Mux7/1 -> Scope/8  "I_Gate"
  Mux6/1 -> Scope/7  "I_Cgd"
  Mux5/1 -> Scope/6  "I_Cgs"
  Mux4/1 -> Scope/5  "I_Cds"
  Mux3/1 -> Scope/4  "I_Channel"
  Mux2/1 -> Scope/3  "Vgd"
  Mux1/1 -> Scope/2  "Vgs"
  Mux/1 -> Scope/1  "Vds"
  [Vdsit] -> Capacitance Calculator/1(Vds)
  Capacitance Calculator/1(Cgs) -> Scope1/1, [Cgst]  "Cgst"
  Capacitance Calculator/2(Cgd) -> Scope1/2, [Cgdt]  "Cgdt"
  Capacitance Calculator/3(Cds) -> Scope1/3, [Cdst]  "Cdst"
  [Cgst] -> Capacitance3/1(c)
  [Cgdt] -> Capacitance1/1(c)
  [Cdst] -> Capacitance2/1(c)
  From39/1 -> Scope2/1, Subtract3/1  "Vds_Top"
  From28/1 -> Scope2/2, Subtract3/2  "Vgs_Top"
  From30/1 -> Gain/1  "I_Cds_Top"
  From31/1 -> Sum3/2, Gain1/1  "I_Cgd_Top"
  From32/1 -> Gain3/1, Sum3/1  "I_Gate_Top"
  From33/1 -> Scope4/1, Subtract4/1  "Vds_Bot"
  From34/1 -> Scope4/2, Subtract4/2  "Vgs_Bot"
  From36/1 -> Gain4/1  "I_Cds_Bot"
  From37/1 -> Sum4/1, Gain5/1  "I_Cgd_Bot"
  From38/1 -> Gain7/1, Sum4/2  "I_Gate_Bot"
  Subtract3/1 -> Scope2/3  "Vgd_Top"
  Subtract4/1 -> Scope4/3  "Vgd_Bot"
  From29/1 -> Saturation9/1  "Idrain_Top"
  From35/1 -> Saturation10/1  "Id_Bot"
  Sum4/1 -> Gain6/1  "I_Cgs_Bot"
  Gain/1 -> Saturation3/1
  Gain1/1 -> Saturation2/1
  Sum3/1 -> Gain2/1  "I_Cgs_Top"
  Gain3/1 -> Saturation7/1
  Gain4/1 -> Saturation4/1
  Gain6/1 -> Saturation6/1
  Gain7/1 -> Saturation8/1
  Gain2/1 -> Saturation1/1
  Saturation1/1 -> Gain10/1, Scope2/7  "I_Cgs"
  Saturation2/1 -> Gain9/1, Scope2/6  "I_Cgd"
  Saturation3/1 -> Gain8/1, Scope2/5  "I_Cds"
  Saturation4/1 -> Scope4/5  "I_Cds"
  Saturation5/1 -> Scope4/6  "I_Cgd"
  Gain5/1 -> Saturation5/1
  Saturation6/1 -> Scope4/7  "I_Cgs"
  Saturation7/1 -> Scope2/8  "I_Gate"
  Saturation8/1 -> Scope4/8  "I_Gate"
  Current Measure3/1(Data) -> To Workspace/1, [Id_Top]
  Saturation9/1 -> Scope5/1, Scope2/4  "Id_top"
  Saturation10/1 -> Scope4/4  "Id_bot"
  Gain8/1 -> Scope5/2  "Icds"
  Gain9/1 -> Scope5/3  "Icgd"
  Gain10/1 -> Scope5/4  "Icgs"
  From40/1 -> Scope5/5  "I_ch"
  From41/1 -> Scope3/2  "Ich_Top"
  From42/1 -> Scope3/4  "Ich_Bot"
  [Vdst] -> Unit Delay1/1, To Workspace1/1
  Unit Delay1/1 -> MATLAB Function/2(Vds)
  Voltage Measure2/1(Data) -> [Vdsit]
  Saturation/1 -> [Idst], To Workspace2/1
  Voltage Measure1/1(Data) -> To Workspace3/1, [Vdst]
  From43/1 -> Scope3/1  "DS Top"
  From44/1 -> Scope3/3  "DS Bot"
  [Vgst] -> Capacitance Calculator/2(Vgs)
  connections:
  Capacitance1/RConn1 -- Cgs/LConn1 -- Cgd/RConn1 -- Capacitance3/LConn1 -- Rg/LConn1 -- Voltage Measure/RConn1
  Simulink-PS Converter/RConn1 -- Controlled Current Source/RConn1
  Current Measure/LConn1 -- Gate/RConn1
  Capacitance1/LConn1 -- Current Measure1/RConn1 -- Cgd/LConn1
  Capacitance2/LConn1 -- Voltage Measure1/RConn1 -- Cds/LConn1 -- Current Measure2/RConn1
  Current Measure3/LConn1 -- Drain/RConn1
  Current Measure2/LConn1 -- Voltage Measure2/RConn1 -- Controlled Current Source/RConn2 -- Rd/RConn1 -- Current Measure1/LConn1
  Lg/LConn1 -- Current Measure/RConn1
  Rss/LConn1 -- SS/RConn1
  Lss/RConn1 -- Ls/LConn1 -- Cds/RConn1 -- Voltage Measure1/RConn2 -- Capacitance2/RConn1 -- Controlled Current Source/LConn1 -- Voltage Measure2/RConn2 -- Cgs/RConn1 -- Capacitance3/RConn1 -- Voltage Measure/RConn2
  Source/RConn1 -- Rs/RConn1
  Ld/RConn1 -- Rd/LConn1
  Lss/LConn1 -- Rss/RConn1
  Rs/LConn1 -- Ls/RConn1
  Current Measure3/RConn1 -- Ld/LConn1
  Rg/RConn1 -- Lg/RConn1

== system InverterModel/GAN HALF BRDIGE LEG2/Voltage Measure3 ==
  PS-Simulink Converter2 : nesl_utility/PS-Simulink Converter  PhysicalDomain=network_engine_domain  SubClassName=ps_output  LeftPortType=input  RightPortType=output  PseudoPeriodic=off  Frequencies=[]  Unit=1  AffineConversion=off
  Voltage Sensor3 : fl_lib/Electrical/Electrical Sensors/Voltage Sensor
  V+ : PMIOPort  Port=1  Side=Right
  V- : PMIOPort  Port=2  Side=Right
  Data : Outport
  wires:
  PS-Simulink Converter2/1 -> Data/1
  connections:
  Voltage Sensor3/LConn1 -- V+/RConn1
  Voltage Sensor3/RConn2 -- V-/RConn1
  PS-Simulink Converter2/LConn1 -- Voltage Sensor3/RConn1

== system InverterModel/GAN HALF BRDIGE LEG2/Voltage Measure6 ==
  PS-Simulink Converter2 : nesl_utility/PS-Simulink Converter  PhysicalDomain=network_engine_domain  SubClassName=ps_output  LeftPortType=input  RightPortType=output  PseudoPeriodic=off  Frequencies=[]  Unit=1  AffineConversion=off
  Voltage Sensor3 : fl_lib/Electrical/Electrical Sensors/Voltage Sensor
  V+ : PMIOPort  Port=1  Side=Right
  V- : PMIOPort  Port=2  Side=Right
  Data : Outport
  wires:
  PS-Simulink Converter2/1 -> Data/1
  connections:
  PS-Simulink Converter2/LConn1 -- Voltage Sensor3/RConn1
  Voltage Sensor3/RConn2 -- V-/RConn1
  Voltage Sensor3/LConn1 -- V+/RConn1

== system InverterModel/Gate Driver/Rate Limiter2 ==
  Inp : Inport
  Constant2 : Constant  Value=(VpulseMax - VpulseMin)/1e-9
  Constant3 : Constant  Value=(VpulseMin - VpulseMax)/1e-9
  Rate Limiter Dynamic : simulink/Discontinuities/Rate Limiter Dynamic
  Outp : Outport
  wires:
  Constant3/1 -> Rate Limiter Dynamic/3
  Constant2/1 -> Rate Limiter Dynamic/1
  Inp/1 -> Rate Limiter Dynamic/2
  Rate Limiter Dynamic/1 -> Outp/1

== system InverterModel/Gate Driver1/Rate Limiter2 ==
  Inp : Inport
  Constant2 : Constant  Value=(VpulseMax - VpulseMin)/1e-9
  Constant3 : Constant  Value=(VpulseMin - VpulseMax)/1e-9
  Rate Limiter Dynamic : simulink/Discontinuities/Rate Limiter Dynamic
  Outp : Outport
  wires:
  Rate Limiter Dynamic/1 -> Outp/1
  Inp/1 -> Rate Limiter Dynamic/2
  Constant2/1 -> Rate Limiter Dynamic/1
  Constant3/1 -> Rate Limiter Dynamic/3

== system InverterModel/Gate Driver2/Rate Limiter2 ==
  Inp : Inport
  Constant2 : Constant  Value=(VpulseMax - VpulseMin)/1e-9
  Constant3 : Constant  Value=(VpulseMin - VpulseMax)/1e-9
  Rate Limiter Dynamic : simulink/Discontinuities/Rate Limiter Dynamic
  Outp : Outport
  wires:
  Rate Limiter Dynamic/1 -> Outp/1
  Inp/1 -> Rate Limiter Dynamic/2
  Constant2/1 -> Rate Limiter Dynamic/1
  Constant3/1 -> Rate Limiter Dynamic/3
